simulink model "control_requirement"  (R2021b)
settings: Solver=VariableStepAuto  StartTime=0.0  StopTime=inf  RelTol=1e-3
undefined symbols (not defined in the file): v_max
libraries: simulink x2
settings Model: Creator=matas  LastModifiedBy=matas

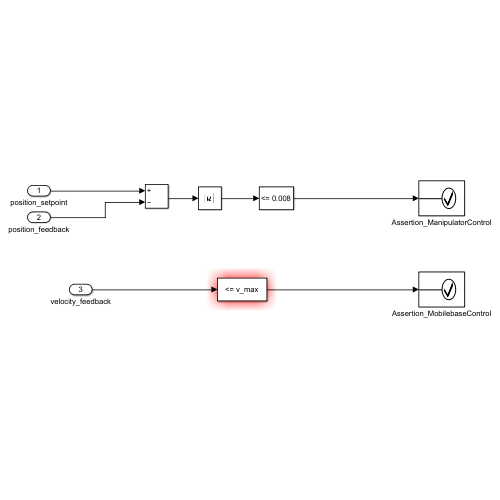
[thumbnail: Simulink's stored preview of the top-level diagram]
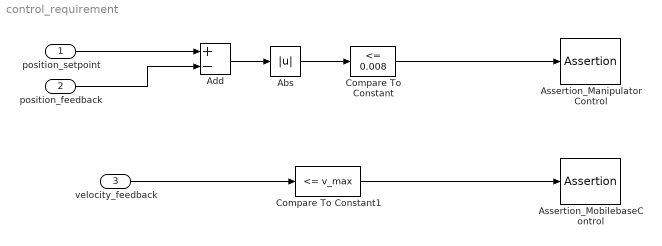
== system control_requirement ==
  position_setpoint : Inport
  position_feedback : Inport  Port=2
  velocity_feedback : Inport  Port=3
  Abs : Abs
  Add : Sum  Inputs=+-
  Assertion_ManipulatorControl : Assertion  StopWhenAssertionFail=off
  Assertion_MobilebaseControl : Assertion  StopWhenAssertionFail=off
  Compare To Constant : simulink/Logic and Bit Operations/Compare To Constant  relop=<=  const=0.008  OutDataTypeStr=boolean
  Compare To Constant1 : simulink/Logic and Bit Operations/Compare To Constant  relop=<=  const=v_max  OutDataTypeStr=boolean
  wires:
  position_feedback/1 -> Add/2
  position_setpoint/1 -> Add/1
  Add/1 -> Abs/1
  Abs/1 -> Compare To Constant/1
  Compare To Constant/1 -> Assertion_ManipulatorControl/1
  velocity_feedback/1 -> Compare To Constant1/1
  Compare To Constant1/1 -> Assertion_MobilebaseControl/1
